simulink model "test1"  (R2018a)
settings: Solver=FixedStepAuto  StartTime=0.0  StopTime=4  FixedStep=0.001  RelTol=1e-3
undefined symbols (not defined in the file): C, h, K, M1, z1, z2
settings Model: Creator=25593  LastModifiedBy=25593

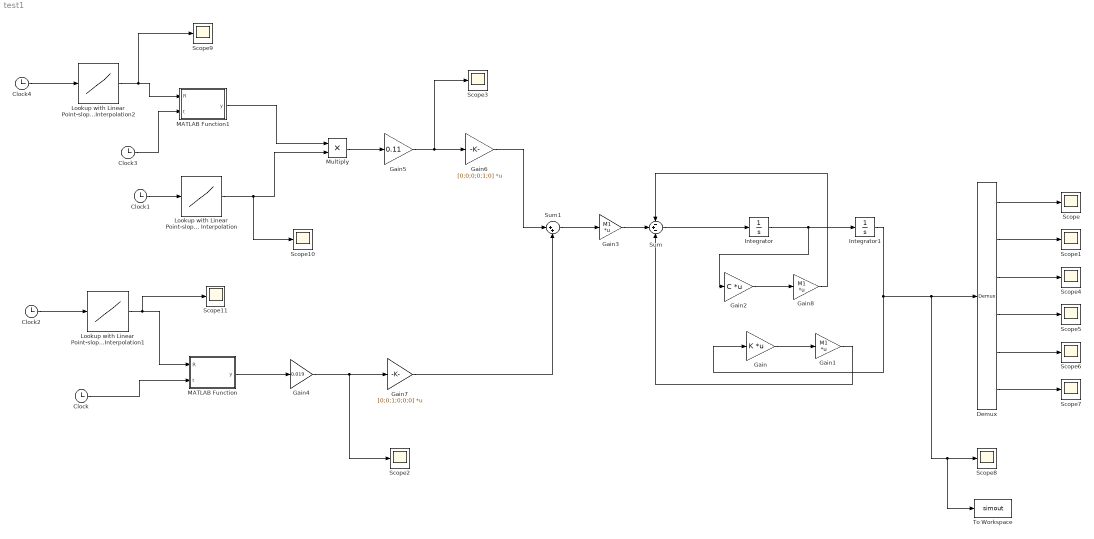
== system test1 ==
  Clock{,1..4} (5 alike) : Clock
  Demux : Demux  Outputs=6
  Gain : Gain  Gain=K  Multiplication=Matrix(K*u)
  Gain1 : Gain  Gain=M1  Multiplication=Matrix(K*u)
  Gain2 : Gain  Gain=C  Multiplication=Matrix(K*u)
  Gain3 : Gain  Gain=M1  Multiplication=Matrix(K*u)
  Gain4 : Gain  Gain=0.019
  Gain5 : Gain  Gain=0.11
  Gain6 : Gain  Gain=[0;0;0;0;1;0]  Multiplication=Matrix(K*u)
  Gain7 : Gain  Gain=[0;0;1;0;0;0]  Multiplication=Matrix(K*u)
  Gain8 : Gain  Gain=M1  Multiplication=Matrix(K*u)
  Integrator : Integrator  InitialCondition=[0;0;0;0;0;0]
  Integrator1 : Integrator  InitialCondition=[0;0;0;0;0;0]
  Lookup with Linear Point-slope Interpolation : Lookup_n-D  NumberOfTableDimensions=1  BreakpointsForDimension1=h  Table=z1  InternalRulePriority=Speed  RndMeth=Simplest  InputSameDT=on
  Lookup with Linear Point-slope Interpolation1 : Lookup_n-D  NumberOfTableDimensions=1  BreakpointsForDimension1=h  Table=z2  InternalRulePriority=Speed  RndMeth=Simplest  InputSameDT=on
  Lookup with Linear Point-slope Interpolation2 : Lookup_n-D  NumberOfTableDimensions=1  BreakpointsForDimension1=h  Table=z2  InternalRulePriority=Speed  RndMeth=Simplest  InputSameDT=on
  MATLAB Function : MATLAB Function  TreatAsAtomicUnit=on
  MATLAB Function1 : MATLAB Function  TreatAsAtomicUnit=on
  Multiply : Product
  Scope{,1..11} (12 alike) : Scope
  Sum : Sum  Inputs=-+-
  Sum1 : Sum  Inputs=|++
  To Workspace : ToWorkspace  VariableName=simout  SampleTime=-1
      settings: Save2DSignal=2-D array (concatenate along first dimension)
  wires:
  Sum/1 -> Integrator/1
  Integrator/1 -> Gain2/1, Integrator1/1
  Gain/1 -> Gain1/1
  Gain1/1 -> Sum/3
  Gain3/1 -> Sum/2
  Clock1/1 -> Lookup with Linear Point-slope Interpolation/1
  Clock2/1 -> Lookup with Linear Point-slope Interpolation1/1
  Clock/1 -> MATLAB Function/2(t)
  Lookup with Linear Point-slope Interpolation1/1 -> Scope11/1, MATLAB Function/1(R)
  MATLAB Function/1(y) -> Gain4/1
  Gain4/1 -> Scope2/1, Gain7/1
  Clock3/1 -> MATLAB Function1/2(t)
  Clock4/1 -> Lookup with Linear Point-slope Interpolation2/1
  Lookup with Linear Point-slope Interpolation2/1 -> Scope9/1, MATLAB Function1/1(R)
  MATLAB Function1/1(y) -> Multiply/1
  Lookup with Linear Point-slope Interpolation/1 -> Scope10/1, Multiply/2
  Multiply/1 -> Gain5/1
  Gain5/1 -> Scope3/1, Gain6/1
  Gain6/1 -> Sum1/1
  Gain7/1 -> Sum1/2
  Sum1/1 -> Gain3/1
  Gain2/1 -> Gain8/1
  Gain8/1 -> Sum/1
  Demux/1 -> Scope/1
  Demux/2 -> Scope1/1
  Demux/3 -> Scope4/1
  Demux/4 -> Scope5/1
  Demux/5 -> Scope6/1
  Demux/6 -> Scope7/1
  Integrator1/1 -> To Workspace/1, Scope8/1, Demux/1, Gain/1

== matlab function test1/MATLAB Function1 ==
  data: R input; y output; t input
function y = fcn(R,t)
y=sin(2*R*2*pi*t/60)

== matlab function test1/MATLAB Function ==
  data: R input; y output; t input
function y = fcn(R,t)
w=R*2*pi/60
y=w*w*cos(2*w*t)
